simulink model "compacaracao"  (R2012b)
settings: Solver=ode3  StartTime=0.0  StopTime=2  FixedStep=1e-4/3  RelTol=1e-3
undefined symbols (not defined in the file or in its folder): SS
libraries: simulink x4, Encoder x2
settings Model: Creator=Juliano  LastModifiedBy=Juliano

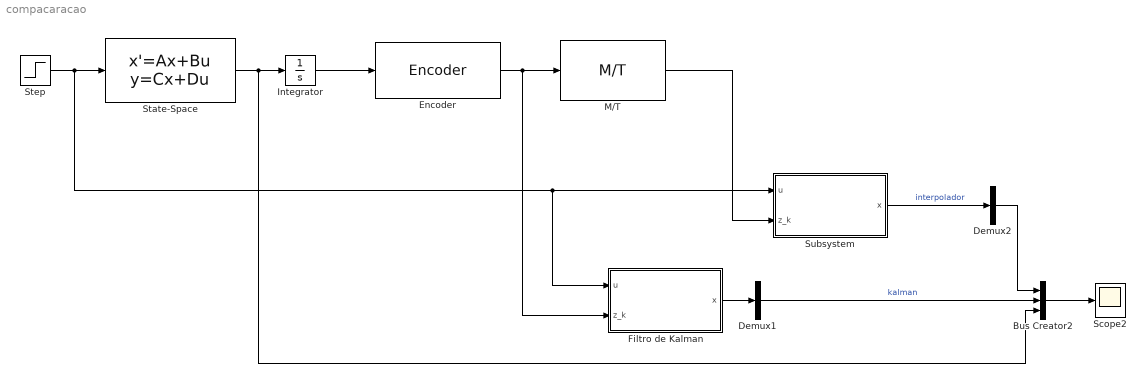
== system compacaracao ==
  Bus Creator2 : BusCreator  Inputs=3
  Demux1 : Demux  Outputs=3
  Demux2 : Demux  Outputs=3
  Encoder : Encoder/Encoder  Nr=10
  Filtro de Kalman : Subsystem
  Integrator : Integrator
  M/T : Encoder/M//T  Ts=0.02
  Scope2 : Scope
      settings: ShowLegends=on  TimeRange=0.0004368562041504875  YMin=5803.198494476836  YMax=5816.985142638738
  State-Space : StateSpace  A=SS.a  B=SS.b  C=SS.c  D=SS.d
  Step : Step  Time=0  After=12  SampleTime=0
  Subsystem : Subsystem
  wires:
  Step/1 -> Subsystem/1(u), Filtro de Kalman/1(u), State-Space/1
  State-Space/1 -> Bus Creator2/3, Integrator/1
  Integrator/1 -> Encoder/1
  Encoder/1 -> Filtro de Kalman/2(z_k), M/T/1
  M/T/1 -> Subsystem/2(z_k)
  Subsystem/1(x) -> Demux2/1  "interpolador"
  Demux2/2 -> Bus Creator2/1
  Bus Creator2/1 -> Scope2/1
  Filtro de Kalman/1(x) -> Demux1/1
  Demux1/2 -> Bus Creator2/2  "kalman"

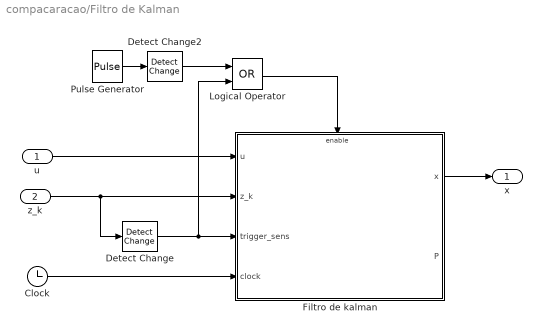
== system compacaracao/Filtro de Kalman ==
  u : Inport
  z_k : Inport  Port=2
  Clock : Clock
  Detect Change : simulink/Logic and Bit Operations/Detect Change  vinit=0  InputProcessing=Inherited  OutDataTypeStr=boolean
  Detect Change2 : simulink/Logic and Bit Operations/Detect Change  vinit=0  InputProcessing=Inherited  OutDataTypeStr=boolean
  Filtro de kalman : Subsystem
  Logical Operator : Logic  Operator=OR  AllPortsSameDT=off  OutDataTypeStr=boolean
  Pulse Generator : DiscretePulseGenerator  PulseType=Time based  Period=0.0004  PulseWidth=50
  x : Outport
  wires:
  Clock/1 -> Filtro de kalman/4(clock)
  Filtro de kalman/1(x) -> x/1
  Logical Operator/1 -> Filtro de kalman/Enable
  z_k/1 -> Detect Change/1, Filtro de kalman/2("z_k ")
  u/1 -> Filtro de kalman/1(u)
  Detect Change/1 -> Logical Operator/2, Filtro de kalman/3(trigger_sens)
  Detect Change2/1 -> Logical Operator/1
  Pulse Generator/1 -> Detect Change2/1

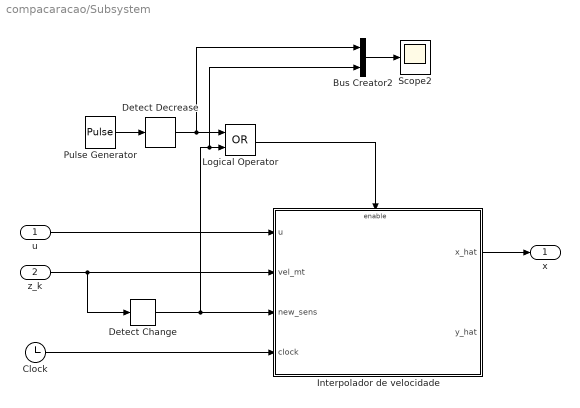
== system compacaracao/Subsystem ==
  u : Inport
  z_k : Inport  Port=2
  Bus Creator2 : BusCreator  Inputs=2
  Clock : Clock
  Detect Change : simulink/Logic and Bit Operations/Detect Change  vinit=0  InputProcessing=Inherited  OutDataTypeStr=boolean
  Detect Decrease : simulink/Logic and Bit Operations/Detect Decrease  vinit=0.0  InputProcessing=Inherited  OutDataTypeStr=boolean
  Interpolador de velocidade : Subsystem
  Logical Operator : Logic  Operator=OR  AllPortsSameDT=off  OutDataTypeStr=boolean
  Pulse Generator : DiscretePulseGenerator  PulseType=Time based  Period=0.0004  PulseWidth=50
  Scope2 : Scope
      settings: ShowLegends=on  YMin=-1  YMax=1.5  SaveName=ScopeData2
  x : Outport
  wires:
  z_k/1 -> Detect Change/1, Interpolador de velocidade/2(vel_mt)
  Interpolador de velocidade/1(x_hat) -> x/1
  u/1 -> Interpolador de velocidade/1(u)
  Clock/1 -> Interpolador de velocidade/4(clock)
  Logical Operator/1 -> Interpolador de velocidade/Enable
  Detect Change/1 -> Bus Creator2/2, Logical Operator/2, Interpolador de velocidade/3(new_sens)
  Detect Decrease/1 -> Logical Operator/1, Bus Creator2/1
  Pulse Generator/1 -> Detect Decrease/1
  Bus Creator2/1 -> Scope2/1

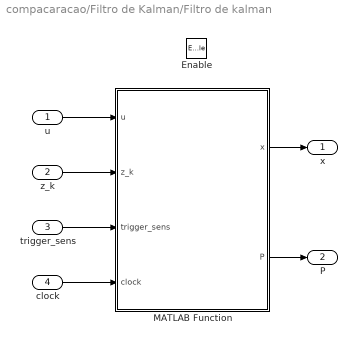
== system compacaracao/Filtro de Kalman/Filtro de kalman ==
  u : Inport
  "z_k " : Inport  Port=2
  trigger_sens : Inport  Port=3
  clock : Inport  Port=4
  Enable : EnablePort
  MATLAB Function : MATLAB Function  TreatAsAtomicUnit=on
  x : Outport
  P : Outport  Port=2
  wires:
  "z_k "/1 -> MATLAB Function/2(z_k)
  clock/1 -> MATLAB Function/4(clock)
  u/1 -> MATLAB Function/1(u)
  trigger_sens/1 -> MATLAB Function/3(trigger_sens)
  MATLAB Function/2(P) -> P/1
  MATLAB Function/1(x) -> x/1

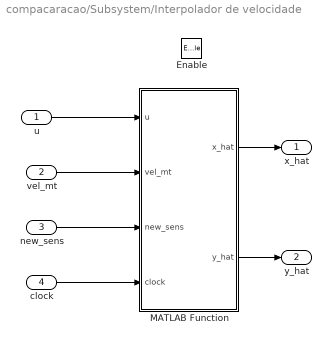
== system compacaracao/Subsystem/Interpolador de velocidade ==
  u : Inport
  vel_mt : Inport  Port=2
  new_sens : Inport  Port=3
  clock : Inport  Port=4
  Enable : EnablePort
  MATLAB Function : MATLAB Function  TreatAsAtomicUnit=on
  x_hat : Outport
  y_hat : Outport  Port=2
  wires:
  new_sens/1 -> MATLAB Function/3(new_sens)
  clock/1 -> MATLAB Function/4(clock)
  vel_mt/1 -> MATLAB Function/2(vel_mt)
  u/1 -> MATLAB Function/1(u)
  MATLAB Function/1(x_hat) -> x_hat/1
  MATLAB Function/2(y_hat) -> y_hat/1

== matlab function compacaracao/Subsystem/Interpolador de velocidade/MATLAB Function ==
  data: u input; x_hat output; vel_mt input; new_sens input; clock input; y_hat output
function [x_hat,y_hat] = fcn(u, vel_mt, new_sens, clock)

    %#codegen
    persistent x;
    persistent t;
    persistent t_sens;
    persistent C;
    persistent D;

    if(isempty(x))
        x = [0 ; 0; 0];
        t = 0;
        t_sens = t;
        C = [0 1 0];
        D = 0;
    end

     if(new_sens == 1)
        x = [x(1) vel_mt x(3)]';
        t_sens = clock;
     else
        deltaT = clock-max(t,t_sens);
        A = [1-3588*deltaT -45060*deltaT 0; deltaT 1 0; 0 deltaT 1];
        B = [2.899e7*deltaT; 0; 0];
        x = A*x+B*u;
        t = clock;
    end
    
    x_hat = x;
    y_hat = C*x+D*u;
end

== matlab function compacaracao/Filtro de Kalman/Filtro de kalman/MATLAB Function ==
  data: u input; z_k input; x output; trigger_sens input; P output; clock input
function [x,P] = fcn(u, z_k, trigger_sens, clock)
%#codegen

persistent t_old;
persistent x_posteriori_old;
persistent P_posteriori_old;

if( isempty(t_old) || isempty(x_posteriori_old) || isempty(P_posteriori_old) )
    t_old = 0;
    x_posteriori_old = [0 0 0]';
    P_posteriori_old = [10 0 0; 0 10 0; 0 0 10];
end


deltaT = clock - t_old;
F = [1-3588*deltaT -45060*deltaT 0 ; deltaT 1 0 ; 0 deltaT 1];
B = [2.899e7*deltaT ; 0 ; 0];
H = [0 0 1];
Q = eye(3)*0.6;
R = eye(1)*0.2;

% Previsão
x_priori = F * x_posteriori_old + B*u;
P_priori = F * P_posteriori_old * F' + Q;

% Atualização
if(trigger_sens == 1)
    y_tilde = z_k - H * x_priori;
    S = H * P_priori * H' + R;
    K = P_priori * H' / S;
    x_posteriori = x_priori + K * y_tilde;
    P_posteriori = (eye(size(K*H)) * K * H) * P_priori;
else
    x_posteriori = x_priori;
    P_posteriori = P_priori;
end

x = x_posteriori;
P = P_posteriori;

x_posteriori_old = x_posteriori;
P_posteriori_old = P_posteriori;
t_old = clock;
